simulink model "yam"  (R2014b)
settings: Solver=ode4  StartTime=0.0  StopTime=10  FixedStep=0.01  RelTol=1e-3
settings Model: Creator=Abhiram  LastModifiedBy=Markus

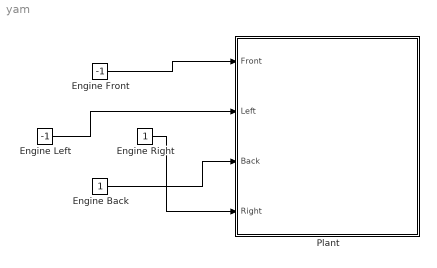
== system yam ==
  Engine Back : Constant
  Engine Front : Constant  Value=-1
  Engine Left : Constant  Value=-1
  Engine Right : Constant
  Plant : Subsystem
  wires:
  Engine Front/1 -> Plant/1(Front)
  Engine Left/1 -> Plant/2(Left)
  Engine Back/1 -> Plant/3(Back)
  Engine Right/1 -> Plant/4(Right)

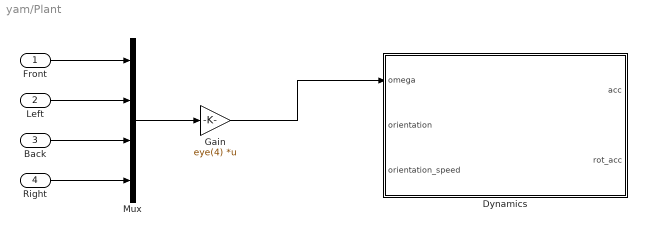
== system yam/Plant ==
  Front : Inport
  Left : Inport  Port=2
  Back : Inport  Port=3
  Right : Inport  Port=4
  Dynamics : MATLAB Function  TreatAsAtomicUnit=on
  Gain : Gain  Gain=eye(4)  Multiplication=Matrix(K*u)
  Mux : Mux
  wires:
  Gain/1 -> Dynamics/1(omega)
  Mux/1 -> Gain/1
  Front/1 -> Mux/1
  Left/1 -> Mux/2
  Back/1 -> Mux/3
  Right/1 -> Mux/4

== matlab function yam/Plant/Dynamics ==
  data: omega input; acc output; rot_acc output; orientation input; orientation_speed input
function [acc, rot_acc] = fcn(omega, orientation, orientation_speed)

mass = 0.027;
gravity = [0 0 -9.81]';
Ixx = 1;
Iyy = 1;
Izz = 1;

Im = diag([Ixx, Iyy, Izz]);


%voltagte to thrust
omega = omega .* 1;

%voltage to torque
vtt = 1;

F = [0 0 sum(omega)]';
R = Quaternion(orientation(1), orientation(2), orientation(3)).getRotationMatrix();
acc = gravity + R * F / mass;




rot_acc = 






end
